simulink model "Recorrer_1_Baldosa"  (R2024b)
settings: Solver=FixedStepDiscrete  StartTime=0.0  StopTime=inf  FixedStep=0.01  RelTol=1e-3  EnableMultiTasking=on
settings Model: Creator=Chenfu  LastModifiedBy=Chenfu

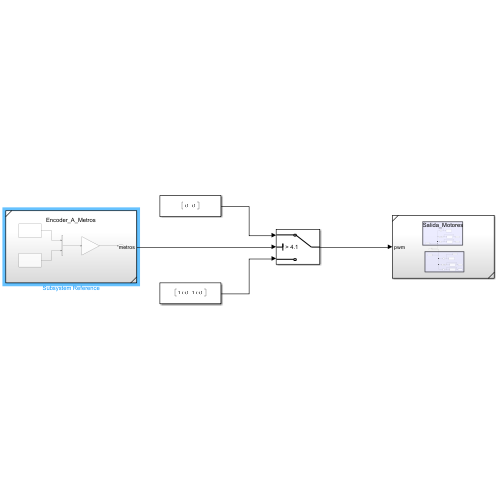
[thumbnail: Simulink's stored preview of the top-level diagram]
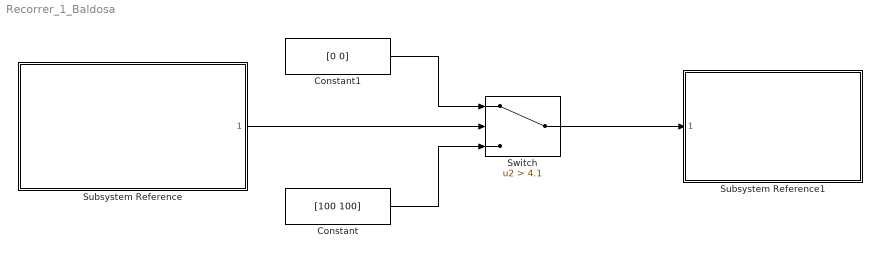
== system Recorrer_1_Baldosa ==
  Constant : Constant  Value=[100 100]  SampleTime=-1
  Constant1 : Constant  Value=[0 0]  SampleTime=-1
  Subsystem Reference : Subsystem  ReferencedSubsystem=Encoder_A_Metros
  Subsystem Reference1 : Subsystem  ReferencedSubsystem=Salida_Motores
  Switch : Switch  Criteria=u2 > Threshold  Threshold=4.1  SaturateOnIntegerOverflow=off  InputSameDT=off
  wires:
  Constant1/1 -> Switch/1
  Constant/1 -> Switch/3
  Subsystem Reference/1 -> Switch/2
  Switch/1 -> Subsystem Reference1/1
